simulink model "untitled"  (R2021a)
settings: Solver=VariableStepAuto  StartTime=0.0  StopTime=10.0  RelTol=1e-3
model workspace (MAT data in the model file):
  phi_dot = Simulink.Signal
  phi_dot.DataType = 'auto'
  phi_dot.Dimensions = 4
  phi_dot.DimensionsMode = 'auto'
  phi_dot.Complexity = 'auto'
  phi_dot.SampleTime = -1
  phi_dot.SamplingMode = 'auto'
  phi_dot.InitialValue = '0.1'
settings Model: Creator=ASUS  LastModifiedBy=ASUS

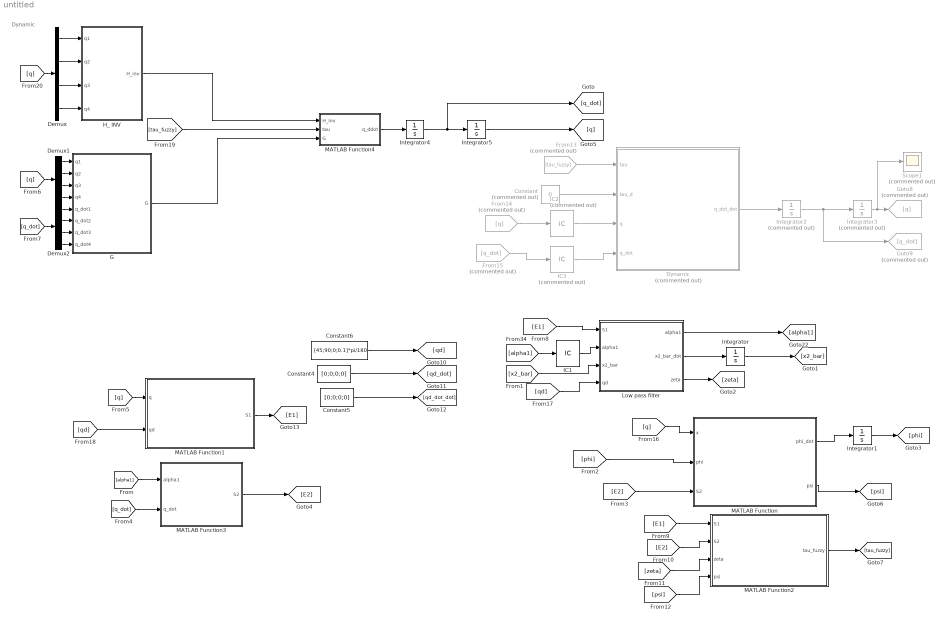
== system untitled ==
  note: Dynamic
  Constant : Constant  Commented=on  Value=0
  Constant4 : Constant  Value=[0;0;0;0]
  Constant5 : Constant  Value=[0;0;0;0]
  Constant6 : Constant  Value=[45;90;0;0.1]*pi/180
  Demux : Demux
  Demux1 : Demux
  Demux2 : Demux
  Dynamic : MATLAB Function  Commented=on  TreatAsAtomicUnit=on
  From13 : From  Commented=on  GotoTag=tau_fuzzy
  From14 : From  Commented=on  GotoTag=q
  From15 : From  Commented=on  GotoTag=q_dot
  G : MATLAB Function  TreatAsAtomicUnit=on
  Goto8 : Goto  Commented=on  GotoTag=q
  Goto9 : Goto  Commented=on  GotoTag=q_dot
  H_ INV : MATLAB Function  TreatAsAtomicUnit=on
  IC1 : InitialCondition  Value=[0.01;0.01;0.01;0.01]
  IC2 : InitialCondition  Commented=on  Value=[0.1; 0.1; 0.1; 0.1]
  IC3 : InitialCondition  Commented=on  Value=[0.1; 0.1; 0.1; 0.1]
  Integrator : Integrator  InitialCondition=zeros(4,1)
  Integrator1 : Integrator  InitialCondition=zeros(4,1)
  Integrator2 : Integrator  Commented=on  InitialCondition=[0.1; 0.1; 0.1; 0.1]
  Integrator3 : Integrator  Commented=on  InitialCondition=[0.1; 0.1; 0.1; 0.1]
  Integrator4 : Integrator  InitialCondition=[0.1; 0.1; 0.1; 0.1]
  Integrator5 : Integrator  InitialCondition=[0.1; 0.1; 0.1; 0.1]
  Low pass filter : MATLAB Function  TreatAsAtomicUnit=on
  MATLAB Function : MATLAB Function  TreatAsAtomicUnit=on
  MATLAB Function1 : MATLAB Function  TreatAsAtomicUnit=on
  MATLAB Function2 : MATLAB Function  TreatAsAtomicUnit=on
  MATLAB Function3 : MATLAB Function  TreatAsAtomicUnit=on
  MATLAB Function4 : MATLAB Function  TreatAsAtomicUnit=on
  Scope1 : Scope  Commented=on
  wires:
  Low pass filter/2(x2_bar_dot) -> Integrator/1
  Integrator/1 -> [x2_bar]
  [x2_bar] -> Low pass filter/3(x2_bar)
  Low pass filter/3(zeta) -> [zeta]
  Integrator1/1 -> [phi]
  [E1] -> Low pass filter/1(S1)
  [E2] -> MATLAB Function/3(S2)
  [E2] -> MATLAB Function2/2(S2)
  [E1] -> MATLAB Function2/1(S1)
  [zeta] -> MATLAB Function2/3(zeta)
  MATLAB Function/2(psi) -> [psi]
  [psi] -> MATLAB Function2/4(psi)
  MATLAB Function2/1(tau_fuzzy) -> [tau_fuzzy]
  From13/1 -> Dynamic/1(tau)
  Constant/1 -> Dynamic/2(tau_d)
  Dynamic/1(q_dot_dot) -> Integrator2/1
  Integrator2/1 -> Goto9/1, Integrator3/1
  Integrator3/1 -> Scope1/1, Goto8/1
  Constant5/1 -> [qd_dot_dot]
  Constant4/1 -> [qd_dot]
  Constant6/1 -> [qd]
  [q] -> MATLAB Function/1(x)
  [qd] -> Low pass filter/4(qd)
  MATLAB Function1/1(S1) -> [E1]
  [q] -> MATLAB Function1/1(q)
  [qd] -> MATLAB Function1/2(qd)
  Low pass filter/1(alpha1) -> [alpha1]
  [alpha1] -> IC1/1
  IC1/1 -> Low pass filter/2("alpha1 ")
  MATLAB Function3/1(S2) -> [E2]
  [alpha1] -> MATLAB Function3/1(alpha1)
  [q_dot] -> MATLAB Function3/2(q_dot)
  [phi] -> MATLAB Function/2(phi)
  From14/1 -> IC2/1
  IC2/1 -> Dynamic/3(q)
  From15/1 -> IC3/1
  IC3/1 -> Dynamic/4(q_dot)
  [q] -> Demux/1
  Demux2/4 -> G/8(q_dot4)
  [q_dot] -> Demux2/1
  Demux1/1 -> G/1(q1)
  Demux1/3 -> G/3(q3)
  Demux1/4 -> G/4(q4)
  Demux2/2 -> G/6(q_dot2)
  Demux2/3 -> G/7(q_dot3)
  H_ INV/1(H_inv) -> MATLAB Function4/1(H_inv)
  [q] -> Demux1/1
  Demux/1 -> H_ INV/1(q1)
  Demux/2 -> H_ INV/2(q2)
  Demux1/2 -> G/2(q2)
  Demux/3 -> H_ INV/3(q3)
  Demux/4 -> H_ INV/4(q4)
  G/1(G) -> MATLAB Function4/3(G)
  [tau_fuzzy] -> MATLAB Function4/2(tau)
  Demux2/1 -> G/5(q_dot1)
  MATLAB Function4/1(q_ddot) -> Integrator4/1
  Integrator4/1 -> Integrator5/1, [q_dot]
  Integrator5/1 -> [q]
  MATLAB Function/1(phi_dot) -> Integrator1/1

== matlab function untitled/MATLAB Function4 ==
  data: H_inv input; tau input; q_ddot output; G input
function q_ddot = fcn(H_inv,tau,G)

q_ddot=H_inv*(tau-G)

== matlab function untitled/Low pass filter ==
  data: S1 input; alpha1 output; alpha1 input; x2_bar input; x2_bar_dot output; zeta output; qd input
function [alpha1,x2_bar_dot,zeta] = fcn(S1,alpha1,x2_bar,qd)
u = 0.1; %filter ceoficient
c1 = 0.1;
x2_bar_dot = -c1*S1+qd;

alpha1 = u*x2_bar + alpha1;

zeta = alpha1 - x2_bar;
end

== matlab function untitled/Dynamic ==
  data: tau input; q_dot_dot output; tau_d input; q input; q_dot input
% function q_dot_dot = fcn(tau,tau_d,q,q_dot)
% 
% q1=q(1);
% q2=q(2);
% q3=q(3);
% q4=q(4);
% 
% q1d=q_dot(1);
% q2d=q_dot(2);
% q3d=q_dot(3);
% q4d=q_dot(4);
% 
% 
% 
% m1=20;
% m2=15;
% m3=15;
% m4=0.5;
% 
% r1 = 0.1;
% r2 = 0.125;
% 
% l1=.2;
% l2=.25;
% 
% Iz1=.27;
% Iz2=.31;
% Iz3=.02;
% Iz4=.0001;
% 
% g=9.81;
% 
% 
% 
% a = Iz1 + ((r1^2)*m1) + ((l1^2)*m2) + ((l1^2)*m3) + ((l1^2)*m4);
% b = Iz2 + Iz3 + Iz4 + ((l2^2)*m3)+ ((l2^2)*m4) + ((r2^2)*m2);
% gamma = (l1*l2*m3)+(l1*l2*m4)+(l1*m2*r2);
% delta = Iz3 + Iz4;
% 
% 
% 
% M=[a+b+(2*gamma*cos(q2)),   b+(gamma*cos(q2))   ,delta, 0  ;
%     b+(gamma*cos(q2))   ,      b                ,delta, 0  ;
%      delta              ,      delta            ,delta, 0  ;
%      0                  ,      0                ,  0  , m4];
% 
% 
% C=[-gamma*sin(q2)*q2d  , -gamma*sin(q2)*(q2d+q1d), 0 , 0 ;
%     gamma*sin(q2)*q1d  ,      0                  , 0 , 0 ;
%      0                 ,      0                  , 0 , 0 ;
%      0                 ,      0                  , 0 , 0];
% 
% 
% G=[ 0 ; 0 ; 0 ; m4*g ];
% 
% 
% q_dot_dot=pinv(M)*(tau + tau_d - (C*q_dot) - G);
% 
% 

% function q_dot_dot = fcn(tau, tau_d, q, q_dot)
% 
% % Ensure input vectors are correctly referenced
% q1 = q(1);
% q2 = q(2);
% q3 = q(3);
% q4 = q(4);
% 
% q1d = q_dot(1);
% q2d = q_dot(2);
% q3d = q_dot(3);
% q4d = q_dot(4);
% 
% % Define constants
% m1 = 20;
% m2 = 15;
% m3 = 15;
% m4 = 0.5;
% 
% r1 = 0.1;
% r2 = 0.125;
% 
% l1 = 0.2;
% l2 = 0.25;
% 
% Iz1 = 0.27;
% Iz2 = 0.31;
% Iz3 = 0.02;
% Iz4 = 0.0001;
% 
% g = 9.81;
% 
% % Calculate terms for the M, C, and G matrices
% a = Iz1 + (r1^2 * m1) + (l1^2 * m2) + (l1^2 * m3) + (l1^2 * m4);
% b = Iz2 + Iz3 + Iz4 + (l2^2 * m3) + (l2^2 * m4) + (r2^2 * m2);
% gamma = (l1 * l2 * m3) + (l1 * l2 * m4) + (l1 * m2 * r2);
% delta = Iz3 + Iz4;
% 
% % Define the mass matrix M
% M = [a + b + 2 * gamma * cos(q2), b + gamma * cos(q2), delta, 0;
%      b + gamma * cos(q2), b, delta, 0;
%      delta, delta, delta, 0;
%      0, 0, 0, m4];
% 
% % Define the Coriolis matrix C
% C = [-gamma * sin(q2) * q2d, -gamma * sin(q2) * (q2d + q1d), 0, 0;
%       gamma * sin(q2) * q1d, 0, 0, 0;
%       0, 0, 0, 0;
%       0, 0, 0, 0];
% 
% % Define the gravity vector G
% G = [0; 0; 0; m4 * g];
% 
% % Calculate q_dot_dot
% q_dot_dot = pinv(M) * (tau + tau_d - (C * q_dot) - G);
% 
% end
function q_dot_dot = fcn(tau, tau_d, q, q_dot)
%#codegen

% Define the output sizes for code generation
coder.varsize('q_dot_dot', [4, 1], [1, 0]);

% Ensure input vectors are correctly referenced
q1 = q(1);
q2 = q(2);
q3 = q(3);
q4 = q(4);

q1d = q_dot(1);
q2d = q_dot(2);
q3d = q_dot(3);
q4d = q_dot(4);

% Define constants
m1 = 20;
m2 = 15;
m3 = 15;
m4 = 0.5;

r1 = 0.1;
r2 = 0.125;

l1 = 0.2;
l2 = 0.25;

Iz1 = 0.27;
Iz2 = 0.31;
Iz3 = 0.02;
Iz4 = 0.0001;

g = 9.81;

% Calculate terms for the M, C, and G matrices
a = Iz1 + (r1^2 * m1) + (l1^2 * m2) + (l1^2 * m3) + (l1^2 * m4);
b = Iz2 + Iz3 + Iz4 + (l2^2 * m3) + (l2^2 * m4) + (r2^2 * m2);
gamma = (l1 * l2 * m3) + (l1 * l2 * m4) + (l1 * m2 * r2);
delta = Iz3 + Iz4;

% Define the mass matrix M
M = [a + b + 2 * gamma * cos(q2), b + gamma * cos(q2), delta, 0;
     b + gamma * cos(q2), b, delta, 0;
     delta, delta, delta, 0;
     0, 0, 0, m4];

% Define the Coriolis matrix C
C = [-gamma * sin(q2) * q2d, -gamma * sin(q2) * (q2d + q1d), 0, 0;
      gamma * sin(q2) * q1d, 0, 0, 0;
      0, 0, 0, 0;
      0, 0, 0, 0];

% Define the gravity vector G
G = [0; 0; 0; m4 * g];

% Add small epsilon to avoid division by zero
epsilon = 1e-6;

% Check for matrix singularity
if cond(M) > 1/epsilon
    warning('Mass matrix is near singular or badly scaled. Results may be inaccurate.');
    M = M + eye(4) * epsilon; % Regularize M to avoid singularity
end

% Calculate q_dot_dot
q_dot_dot = pinv(M) * (tau + tau_d - (C * q_dot) - G);

% Diagnostic print statements (remove or comment out in production)

end

== matlab function untitled/MATLAB Function ==
  data: x input; phi input; phi_dot output size=[4, 1]; S2 input; psi output
function [phi_dot, psi] = fuzz(x, phi, S2)
    % Define constants
    m = 0.1;
    k = 0.1;

    % Define parameters for triangular membership functions
    inputMFParams = {
        {[-0.04 -0.04 -0.03], [-0.04 -0.04 -0.03], [-0.04 -0.04 -0.03], [-0.04 -0.04 -0.03]}, ... % Rule 1
        {[-0.04 -0.03 -0.02], [-0.04 -0.03 -0.02], [-0.04 -0.03 -0.02], [-0.04 -0.03 -0.02]}, ... % Rule 2
        {[-0.03 -0.02 -0.01], [-0.03 -0.02 -0.01], [-0.03 -0.02 -0.01], [-0.03 -0.02 -0.01]}, ... % Rule 3
        {[-0.02 -0.01 0], [-0.02 -0.01 0], [-0.02 -0.01 0], [-0.02 -0.01 0]}                   % Rule 4
    }; % NB, NS, Z, PS, PB

    % Calculate gamma matrix
    gammaMatrix = calculateGammaMatrix(x, inputMFParams);

    % Ensure gammaMatrix is a 4x4 matrix for the calculation
    gammaMatrix = gammaMatrix(1:4, :); 

    % Compute phi_dot
    phi_dot = m * pinv(S2 * gammaMatrix) - 2 * k * phi;

    % Compute psi
    psi = gammaMatrix * phi;
end

% Triangular membership function
function mu = trimf(x, params)
    a = params(1);
    b = params(2);
    c = params(3);
    if x <= a
        mu = 0;
    elseif a < x && x <= b
        mu = (x - a) / (b - a);
    elseif b < x && x <= c
        mu = (c - x) / (c - b);
    else
        mu = 0;
    end
end

% Evaluate gamma values
function gammaMatrix = calculateGammaMatrix(x, inputMFParams)
    N = size(inputMFParams, 1); % Number of rules
    n = size(inputMFParams{1}, 1); % Number of inputs
    product_mu = zeros(N, 1);
    sum_product_mu = 0;
    
    % Evaluate membership functions for each input and each rule
    for i = 1:4
        mu_product = 1;
        for j = 1:4
            mu_product = mu_product * trimf(x(j), inputMFParams{i}{j});
        end
        product_mu(i) = mu_product;
        sum_product_mu = sum_product_mu + mu_product;
    end
    
    % Calculate gamma values
    gamma = product_mu / sum_product_mu;
    
    % Arrange gamma values in a block diagonal matrix
    gammaMatrix = blkdiag(gamma(1), gamma(2), gamma(3), gamma(4));
end
%%%%%%%%%%%%%%%%%%%%%%%%%%%%%%%%%%%%%%%%%%%%%%%
% function [phi_dot, psi] = fuzz(x, phi, S2)
%     % Define constants
%     m = 0.1;
%     k = 0.1;
% 
%     % Define parameters for triangular membership functions
%     inputMFParams = {
%         {[-0.04 -0.04 -0.03], [-0.04 -0.04 -0.03], [-0.04 -0.04 -0.03], [-0.04 -0.04 -0.03]}, ... % Rule 1
%         {[-0.04 -0.03 -0.02], [-0.04 -0.03 -0.02], [-0.04 -0.03 -0.02], [-0.04 -0.03 -0.02]}, ... % Rule 2
%         {[-0.03 -0.02 -0.01], [-0.03 -0.02 -0.01], [-0.03 -0.02 -0.01], [-0.03 -0.02 -0.01]}, ... % Rule 3
%         {[-0.02 -0.01 0], [-0.02 -0.01 0], [-0.02 -0.01 0], [-0.02 -0.01 0]}                   % Rule 4
%     }; % NB, NS, Z, PS, PB
% 
%     % Calculate gamma matrix
%     gammaMatrix = calculateGammaMatrix(x, inputMFParams);
% 
%     % Compute phi_dot
%     phi_dot = m * pinv(S2 * diag(gammaMatrix)) - 2 * k * phi;
% 
%     % Compute psi
%     psi = diag(gammaMatrix) .* phi;
% end
% 
% % Triangular membership function
% function mu = trimf(x, params)
%     a = params(1);
%     b = params(2);
%     c = params(3);
%     if x <= a
%         mu = 0;
%     elseif a < x && x <= b
%         mu = (x - a) / (b - a);
%     elseif b < x && x <= c
%         mu = (c - x) / (c - b);
%     else
%         mu = 0;
%     end
% end
% 
% % Evaluate gamma values
% function gammaMatrix = calculateGammaMatrix(x, inputMFParams)
%     N = size(inputMFParams, 1); % Number of rules
%     n = size(inputMFParams{1}, 1); % Number of inputs
%     product_mu = zeros(N, 1);
%     sum_product_mu = 0;
%     
%     % Evaluate membership functions for each input and each rule
%     for i = 1:N
%         mu_product = 1;
%         for j = 1:n
%             mu_product = mu_product * trimf(x(j), inputMFParams{i}{j});
%         end
%         product_mu(i) = mu_product;
%         sum_product_mu = sum_product_mu + mu_product;
%     end
%     
%     % Calculate gamma values
%     gamma = product_mu / sum_product_mu;
%     
%     % Ensure gammaMatrix is a 4x4 matrix for the calculation
%     gammaMatrix = zeros(4, 4);
%     for i = 1:min(4, length(gamma))
%         gammaMatrix(i, i) = gamma(i);
%     end
% end
%%%%%%%%%%%%%%%%%%%%%%%%%%%%%%%%%%%%%%
% function [phi_dot, psi] = fuzz(x, phi, S2)
%     %#codegen
% 
%     % Define constants
%     m = 0.1;
%     k = 0.1;
% 
%     % Define parameters for triangular membership functions
%     inputMFParams = {
%         {[-0.04 -0.04 -0.03], [-0.04 -0.04 -0.03], [-0.04 -0.04 -0.03], [-0.04 -0.04 -0.03]}, ... % Rule 1
%         {[-0.04 -0.03 -0.02], [-0.04 -0.03 -0.02], [-0.04 -0.03 -0.02], [-0.04 -0.03 -0.02]}, ... % Rule 2
%         {[-0.03 -0.02 -0.01], [-0.03 -0.02 -0.01], [-0.03 -0.02 -0.01], [-0.03 -0.02 -0.01]}, ... % Rule 3
%         {[-0.02 -0.01 0], [-0.02 -0.01 0], [-0.02 -0.01 0], [-0.02 -0.01 0]}                   % Rule 4
%     }; % NB, NS, Z, PS, PB
% 
%     % Calculate gamma matrix
%     gammaMatrix = calculateGammaMatrix(x, inputMFParams);
% 
%     % Ensure gammaMatrix is a 4x1 vector for calculation
%     gammaVector = diag(gammaMatrix);  % Extract the diagonal elements as a vector
% 
%     % Compute phi_dot
%     phi_dot = m * pinv(pinv(S2) * gammaVector) - 2 * k * phi;
% 
%     % Compute psi
%     psi = gammaVector .* phi;
% end
% 
% Triangular membership function

% function phi_dot  = fuzz(x, phi, S2, psi)
% %#codegen
% 
% % Define constants
% m = 0.1;
% k = 0.1;
% 
% % Assert the sizes of the inputs
% assert(all(size(x) == [4, 1]));
% assert(all(size(phi) == [4, 1]));
% assert(isscalar(S2));
% 
% % Predefine the size of the outputs
% phi_dot = zeros(4, 1); % Fixed size output
% psi = zeros(4, 1);     % Fixed size output
% 
% % Define parameters for triangular membership functions
% inputMFParams = {
%     {[-0.04, -0.04, -0.03], [-0.04, -0.04, -0.03], [-0.04, -0.04, -0.03], [-0.04, -0.04, -0.03]}, ... % Rule 1
%     {[-0.04, -0.03, -0.02], [-0.04, -0.03, -0.02], [-0.04, -0.03, -0.02], [-0.04, -0.03, -0.02]}, ... % Rule 2
%     {[-0.03, -0.02, -0.01], [-0.03, -0.02, -0.01], [-0.03, -0.02, -0.01], [-0.03, -0.02, -0.01]}, ... % Rule 3
%     {[-0.02, -0.01,  0.00], [-0.02, -0.01,  0.00], [-0.02, -0.01,  0.00], [-0.02, -0.01,  0.00]}  ... % Rule 4
% }; % NB, NS, Z, PS, PB
% 
% % Calculate gamma values for each input
% gamma1 = calculateGamma(x(1), inputMFParams);
% gamma2 = calculateGamma(x(2), inputMFParams);
% gamma3 = calculateGamma(x(3), inputMFParams);
% gamma4 = calculateGamma(x(4), inputMFParams);
% 
% % Form the gamma matrix
% gammaMatrix = blkdiag(gamma1, gamma2, gamma3, gamma4);
% 
% % Compute phi_dot
% phi_dot = m * pinv(S2 * gammaMatrix) - 2 * k * phi;
% 
% % Compute psi
% psi = gammaMatrix * phi;
% 
% end
% function mu = trimf(x, params)
%     a = params(1);
%     b = params(2);
%     c = params(3);
%     if x <= a
%         mu = 0;
%     elseif a < x && x <= b
%         mu = (x - a) / (b - a);
%     elseif b < x && x <= c
%         mu = (c - x) / (c - b);
%     else
%         mu = 0;
%     end
% end
% 
% % Evaluate gamma values
% function gammaMatrix = calculateGammaMatrix(x, inputMFParams)
%     N = size(inputMFParams, 1); % Number of rules
%     n = size(inputMFParams{1}, 1); % Number of inputs
%     product_mu = zeros(N, 1);
%     sum_product_mu = 0;
% 
%     % Evaluate membership functions for each input and each rule
%     for i = 1:N
%         mu_product = 1;
%         for j = 1:n
%             mu_product = mu_product * trimf(x(j), inputMFParams{i}{j});
%         end
%         product_mu(i) = mu_product;
%         sum_product_mu = sum_product_mu + mu_product;
%     end
%     
%     % Calculate gamma values
%     gamma = product_mu / sum_product_mu;
%     
%     % Ensure gammaMatrix is a 4x4 matrix for the calculation
%     gammaMatrix = zeros(4, 4);
%     for i = 1:min(4, length(gamma))
%         gammaMatrix(i, i) = gamma(i);
%     end
% end
% % % Triangular membership function
% % function mu = trimf(x, params)
% % a = params(1);
% % b = params(2);
% % c = params(3);
% % if x <= a
% %     mu = 0;
% % elseif a < x && x <= b
% %     mu = (x - a) / (b - a);
% % elseif b < x && x <= c
% %     mu = (c - x) / (c - b);
% % else
% %     mu = 0;
% % end
% % end
% % 
% % % Evaluate gamma values for a single input
% % function gamma = calculateGamma(x, inputMFParams)
% % N = size(inputMFParams, 1); % Number of rules
% % product_mu = zeros(N, 1);
% % sum_product_mu = 0;
% % 
% % % Evaluate membership functions for the input
% % for i = 1:N
% %     mu_product = 1;
% %     for j = 1:length(inputMFParams{i})
% %         mu_product = mu_product * trimf(x, inputMFParams{i}{j});
% %     end
% %     product_mu(i) = mu_product;
% %     sum_product_mu = sum_product_mu + mu_product;
% % end
% % 
% % % Calculate gamma values
% % gamma = product_mu / sum_product_mu;
% % 
% % % Ensure gamma is a 4x1 vector for the calculation
% % gamma = diag(gamma);
% % 
% % end

== matlab function untitled/MATLAB Function3 ==
  data: alpha1 input; S2 output; q_dot input
function S2  = error1(alpha1,q_dot)
% 
% S1 = [1;2;3;4];

S2 = q_dot - alpha1;
end

== matlab function untitled/MATLAB Function2 ==
  data: S1 input; tau_fuzzy output; S2 input; zeta input; psi input
function tau_fuzzy = fuzzcon(S1,S2,zeta,psi)
c2 = 0.1;

tau_fuzzy = -c2*S2 - S1 -zeta - psi;

end

== matlab function untitled/MATLAB Function1 ==
  data: S1 output; q input; qd input
function S1  = error1(q,qd)
% alpha1,q_dot
S1 = [1;2;3;4];

% S2 = q_dot - alpha1;
end

== matlab function untitled/G ==
  data: G output; q1 input; q2 input; q3 input; q4 input; q_dot1 input; q_dot2 input; q_dot3 input; q_dot4 input
function G = G_matrix(q1,q2,q3,q4,q_dot1,q_dot2,q_dot3,q_dot4)
m1=10;
m2=5;
m3=3;
m4=3;
l1=0.2;
l2=0.2;
R=0.03;
g=9.81;
G=zeros(4,1);

c112=0.5*l1*l2*(m2*+2*(m3+m4))*sin(q2);
c211=-0.5*l1*l2*(m2*+2*(m3+m4))*sin(q2);
c122=0;

G(1)=2*c112*q_dot1*q_dot2+c122*q_dot2^2;
G(2)=c211*q_dot1^2;
G(3)=-(m3+m4)*g;
G(4)=0;
G=[G(1);G(2);G(3);G(4)];

== matlab function untitled/H_ INV ==
  data: q1 input; q2 input; H_inv output; q3 input; q4 input
function H_inv = H_matrix(q1,q2,q3,q4)
m=[10;5;3;3];
l=[0.2 0.2];
R=0.03;

H=zeros(4,4)
H(1,1)=l(1)^2*m(1)/3 + m(2)*(l(1)^2/3 + l(2)^2 + l(1)*l(2)*cos(q2)) + (m(3)*m(4))*( l(1)^2 + l(2)^2 +2*l(1)*l(2)*cos(q2)) +R^2*m(4)/4;
H(1,2)=m(2)*l(2)^2/3 + m(2)*l(1)*l(2)*cos(q2)/2  + m(3)*l(2)^2 + m(3)*l(1)*l(2)*cos(q2) + m(4)*l(2)^2 + m(4)*l(1)*l(2)*cos(q2) +R^2*m(4)/2;
H(1,3)=0;
H(1,4)= -0.5 * m(4)*R^2;

H(2,1)=m(2)*l(2)^2/3 + m(2)*l(1)*l(2)*cos(q2)/2  + m(3)*l(2)^2 + m(3)*l(1)*l(2)*cos(q2) + m(4)*l(2)^2 + m(4)*l(1)*l(2)*cos(q2) +R^2*m(4)/2;
H(2,2)=l(2)*m(2)/3 + l(2)^2*m(3) + l(2)^2*m(4) + 0.5 * m(4)*R^2
H(2,3)=0
H(2,4)=-0.5 * m(4)*R^2;
 
H(3,1)=0
H(3,2)=0
H(3,3)=m(3)+m(4)
H(3,4)=0


H(4,1)=-0.5 * m(4)*R^2;
H(4,2)=-0.5 * m(4)*R^2;
H(4,4)= 0.5 * m(4)*R^2
H(4,3)=0


H_inv =inv(H) ;
